simulink model "Suspansiyon_Sistemi"  (R2023b)
settings: Solver=VariableStepAuto  StartTime=0.0  StopTime=10.0  RelTol=1e-3
libraries: slpidlib x1
settings Model: Creator=Everest  LastModifiedBy=Everest

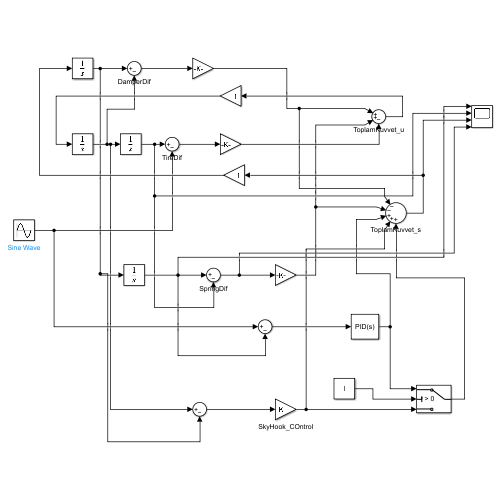
[thumbnail: Simulink's stored preview of the top-level diagram]
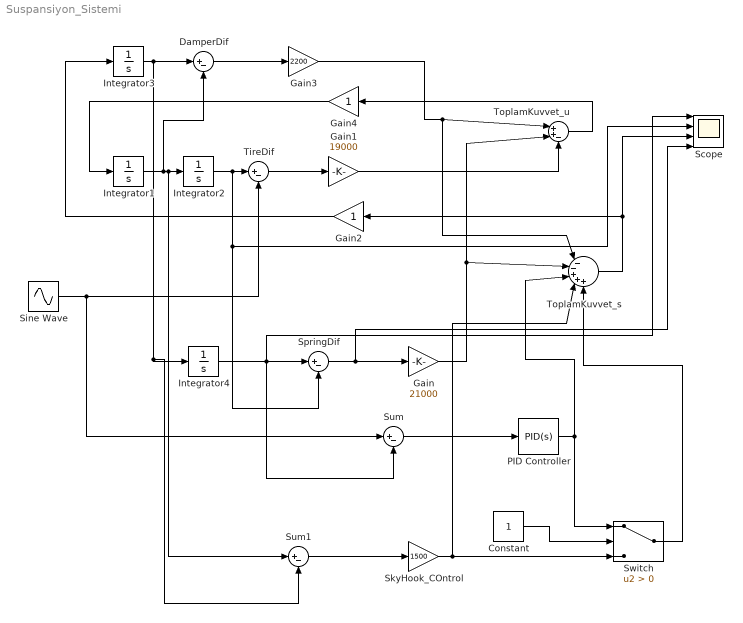
== system Suspansiyon_Sistemi ==
  Constant : Constant
  DamperDif : Sum  Inputs=|+-
  Gain : Gain  Gain=21000
  Gain1 : Gain  Gain=19000
  Gain2 : Gain
  Gain3 : Gain  Gain=2200
  Gain4 : Gain
  Integrator{1..4} (4 alike) : Integrator
  PID Controller : slpidlib/PID Controller  Controller=PID  Form=Parallel  TimeDomain=Continuous-time  UseExternalTs=off  SampleTime=-1  IntegratorMethod=Forward Euler  FilterMethod=Forward Euler  ControllerParametersSource=internal  P=1000  I=50  UseKiTs=off  D=100  N=100  UseFilter=on  TunerSelectOption=Transfer Function Based (PID Tuner App)  InitialConditionSource=internal  InitialConditionForIntegrator=0  InitialConditionForFilter=0  DifferentiatorICPrevScaledInput=0  ExternalReset=none  TrackingMode=off  Kt=1  LimitOutput=off  SatLimitsSource=internal  UpperSaturationLimit=inf  LowerSaturationLimit=-inf  LinearizeAsGain=on  AntiWindupMode=none  Kb=1  LimitIntegrator=off  UpperIntegratorSaturationLimit=inf  LowerIntegratorSaturationLimit=-inf  POutMin=[]  POutMax=[]  IOutMin=[]  IOutMax=[]  DOutMin=[]  DOutMax=[]  NOutMin=[]  NOutMax=[]  SumOutMin=[]  SumOutMax=[]  SaturationOutMin=[]  SaturationOutMax=[]  PParamMin=[]  PParamMax=[]  IParamMin=[]  IParamMax=[]  DParamMin=[]  DParamMax=[]  NParamMin=[]  NParamMax=[]  KbParamMin=[]  KbParamMax=[]  KtParamMin=[]  KtParamMax=[]  KbOutMin=[]  KbOutMax=[]  KtOutMin=[]  KtOutMax=[]  IntegratorOutMin=[]  IntegratorOutMax=[]  FilterOutMin=[]  FilterOutMax=[]  SumI1OutMin=[]  SumI1OutMax=[]  SumI2OutMin=[]  SumI2OutMax=[]  SumI3OutMin=[]  SumI3OutMax=[]  SumI4OutMin=[]  SumI4OutMax=[]  SumDOutMin=[]  SumDOutMax=[]  DifferentiatorOutMin=[]  DifferentiatorOutMax=[]  FilterDiffOutCoefMin=[]  FilterDiffOutCoefMax=[]  ReciprocalOutMin=[]  ReciprocalOutMax=[]  SumDenOutMin=[]  SumDenOutMax=[]  SumNumOutMin=[]  SumNumOutMax=[]  DivideOutMin=[]  DivideOutMax=[]  UdiffTsProdOutMin=[]  UdiffTsProdOutMax=[]  NTsProdOutMin=[]  NTsProdOutMax=[]  UintegralTsProdOutMin=[]  UintegralTsProdOutMax=[]  UngainTsProdOutMin=[]  UngainTsProdOutMax=[]  ClampingZeroOutDataTypeStr=Inherit: Inherit via back propagation  ClampingZeroOutMin=[]  ClampingZeroOutMax=[]  FilterDenConstantOutDataTypeStr=Inherit: Inherit via back propagation  FilterDenConstantOutMin=[]  FilterDenConstantOutMax=[]  PCopyOutDataTypeStr=Inherit: Inherit via back propagation  PCopyOutMin=[]  PCopyOutMax=[]  NCopyOutDataTypeStr=Inherit: Inherit via back propagation  NCopyOutMin=[]  NCopyOutMax=[]  IntegratorContinuousStateAttributes=''  IntegratorStateMustResolveToSignalObject=off  IntegratorRTWStateStorageClass=Auto  FilterContinuousStateAttributes=''  FilterStateMustResolveToSignalObject=off  FilterRTWStateStorageClass=Auto  ParallelPVariant=InternalParameters  IdealPVariant=Disabled  IVariant=InternalParameters  DVariant=InternalParameters  IntegratorVariant=Continuous  SatVariant=Disabled  AWVariant=Passthrough  PCopyVariant=Disabled  TRVariant=Disabled  FdbkBlocksVariant=Forward  IdealPFdbkVariant=Disabled  SatFdbkVariant=Disabled  DerivativeFilterVariant=ContFilter  NVariant=InternalParameters  NCopyVariant=Disabled  FilterICVariant=InternalICsFilter  IntegratorICVariant=InternalICs  ExternalResetVariant=Disabled  TRSumVariant=Passthrough  SumFdbkVariant=Disabled  SumVariant=Sum_PID  TsampFilterVariant=InternalTs  TsampNgainVariant=Passthrough  TsampIntegralVariant=Disabled_SignalSpec  ExternalSaturationOutDataTypeStr=Inherit: Same as second input
  Scope : Scope  NumInputPorts=4
  Sine Wave : Sin  SampleTime=0
  SkyHook_COntrol : Gain  Gain=1500
  SpringDif : Sum  Inputs=|+-
  Sum : Sum  Inputs=|+-
  Sum1 : Sum  Inputs=|+-
  Switch : Switch  Criteria=u2 > Threshold  SaturateOnIntegerOverflow=off  InputSameDT=off
  TireDif : Sum  Inputs=|+-
  ToplamKuvvet_s : Sum  Inputs=|--+++
  ToplamKuvvet_u : Sum  Inputs=|++-
  wires:
  Integrator2/1 -> Scope/2, SpringDif/2, TireDif/1
  TireDif/1 -> Gain1/1
  Integrator1/1 -> Sum1/1, Integrator2/1, DamperDif/2
  Integrator3/1 -> Sum1/2, Integrator4/1, DamperDif/1
  Integrator4/1 -> Scope/1, Sum/2, SpringDif/1
  SpringDif/1 -> Scope/4, Gain/1
  DamperDif/1 -> Gain3/1
  Gain3/1 -> ToplamKuvvet_u/1, ToplamKuvvet_s/1
  Gain1/1 -> ToplamKuvvet_u/3
  Gain/1 -> ToplamKuvvet_s/2, ToplamKuvvet_u/2
  ToplamKuvvet_u/1 -> Gain4/1
  Gain4/1 -> Integrator1/1
  ToplamKuvvet_s/1 -> Scope/3, Gain2/1
  Gain2/1 -> Integrator3/1
  PID Controller/1 -> ToplamKuvvet_s/3, Switch/1
  Sum/1 -> PID Controller/1
  Sum1/1 -> SkyHook_COntrol/1
  SkyHook_COntrol/1 -> Switch/3, ToplamKuvvet_s/4
  Switch/1 -> ToplamKuvvet_s/5
  Constant/1 -> Switch/2
  Sine Wave/1 -> Sum/1, TireDif/2
